simulink model "ACDCMG_sim8"  (R2022a)
settings: Solver=FixedStepAuto  StartTime=0.0  StopTime=0.5  FixedStep=Ts  MaxStep=1e-2  RelTol=1e-3
InitFcn:
  | Set_parameters_R2018
values from neighbouring files (symbols this model uses):
  D_invs = 0.05    [Set_parameters_R2018.m]
  dis11 = 3    [Set_parameters_R2018.m]
  dis12 = 3    [Set_parameters_R2018.m]
  dis2 = 0.2    [Set_parameters_R2018.m]
  dis3 = 0.15    [Set_parameters_R2018.m]
  dis4 = 0.2    [Set_parameters_R2018.m]
  dis5 = 0.25    [Set_parameters_R2018.m]
  dis6 = 0.1    [Set_parameters_R2018.m]
  Fnom = 60    [Set_parameters_R2018.m]
  H_invs = 6    [Set_parameters_R2018.m]
  max_min = 1    [Set_parameters_R2018.m]
  P_Load_3 = S_Load_3* PF_Load_3    (= 7650)    [Set_parameters_R2018.m]
  P_nom_inv = 3e3    (= 3000)    [Set_parameters_R2018.m]
  Pnom_T1 = 1.5e6    (= 1500000)    [Set_parameters_R2018.m]
  Pnom_T2 = 1.5e6    (= 1500000)    [Set_parameters_R2018.m]
  Pnom_T3 = 4e6    (= 4000000)    [Set_parameters_R2018.m]
  Ql_Load_3 = S_Load_3 * sin(acos(PF_Load_3))    [Set_parameters_R2018.m]
  R_Load_9 = (Vnom_prim * 1.35)^2 / P_Load_9    (= 1084.6153125)    [Set_parameters_R2018.m]
  R_Load_DC = Vnom_DC^2/ P_Load_DC    (= 45)    [Set_parameters_R2018.m]
  Rl = 0.17    [Set_parameters_R2018.m]
  Rls = 0.013    [Set_parameters_R2018.m]
  Ts = Ts_Power    (= 6.94444444444e-06)    [Set_parameters_R2018.m]
  Ts_Control = 6*Ts_Power    (= 4.16666666667e-05)    [Set_parameters_R2018.m]
  Ts_Inv = 0.07    [Set_parameters_R2018.m]
  Ts_Power = 1/(24*Fnom)/100    (= 6.94444444444e-06)    [Set_parameters_R2018.m]
  Ts_PV = 0.05    [Set_parameters_R2018.m]
  V1_LL_T3 = 69e3    (= 69000)    [Set_parameters_R2018.m]
  Vmin_mppt = 100    [Set_parameters_R2018.m]
  Vnom_DC = 300    [Set_parameters_R2018.m]
  Vnom_Diesel = 2.4e3    (= 2400)    [Set_parameters_R2018.m]
  Vnom_prim = 13.8e3    (= 13800)    [Set_parameters_R2018.m]
  Vnom_sec = 220    [Set_parameters_R2018.m]
  Vnom_ter_AC_DC = 150    [Set_parameters_R2018.m]
  Xl = 0.3    [Set_parameters_R2018.m]
  Xls = 0.93e-3    (= 0.00093)    [Set_parameters_R2018.m]
undefined symbols (not defined in the file or in its folder): D1, dEgdT, Delta, DiscIntNeverNeededParam, EgRef, fn, gcbh, Ion, k1, Lithium, Rsh_array5pc, sps_rtmsupport, Tref_K, VnInv, VT_ref
libraries: spsCurrentMeasurementLib x40, spsRMSLib x29, spsSeriesRLCBranchLib x23, spsVoltageMeasurementLib x21, spsMeanLib x14, spsThreePhaseVIMeasurementLib x14, powerlib_extras x13, spsThreePhaseSeriesRLCBranchLib x12, spsPower3phInstantaneousLib x10, spsBreakerLib x8, spsControlledVoltageSourceLib x8, spsPowerLib x8
(part 3 of 12)

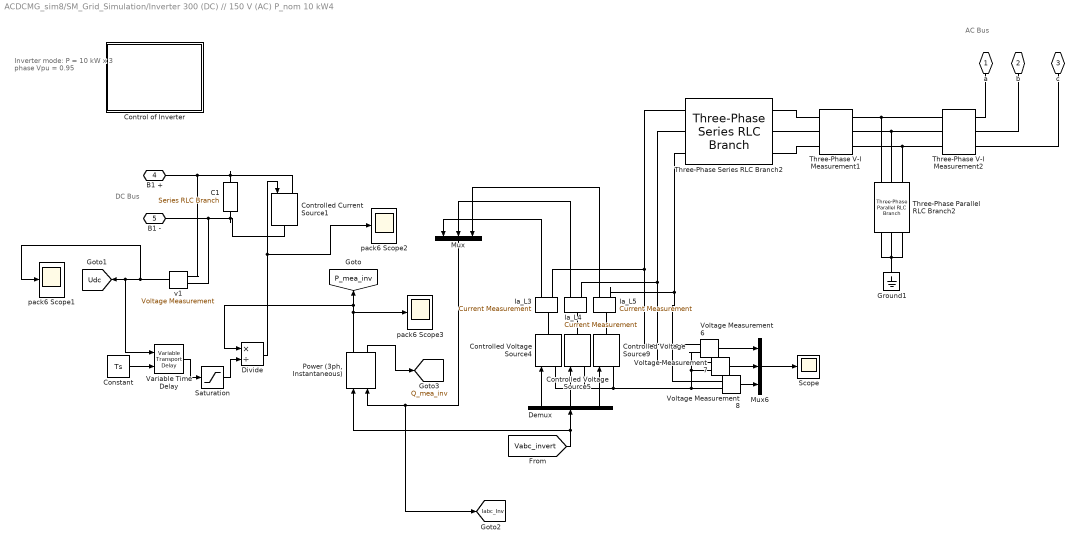
== system ACDCMG_sim8/SM_Grid_Simulation/Inverter 300 (DC) // 150 V (AC) P_nom 10 kW4 ==
  note: DC Bus
  note: AC Bus
  note: Inverter mode:
      |
      | P = 10 kW x 3 phase
      | Vpu = 0.95
  C1 : spsSeriesRLCBranchLib/Series RLC Branch  LConnTagsString=__new0  RConnTagsString=__new0  BranchType=C  Resistance=22.5  Inductance=1e-3  SetiL0=off  InitialCurrent=0  Capacitance=1200e-6  Setx0=on  InitialVoltage=300  Measurements=None
  Constant : Constant  Value=Ts
  Control of Inverter : Subsystem
      mask Display: image('Icons\FPGA.png');
  Controlled Current Source1 : spsControlledCurrentSourceLib/Controlled Current Source  Initialize=on  Source_Type=AC  Amplitude=0  Phase=0  Frequency=0  Measurements=None
  Controlled Voltage Source4 : spsControlledVoltageSourceLib/Controlled Voltage Source  Initialize=off  Source_Type=AC  Amplitude=VnInv*sqrt(2)  Phase=0  Frequency=fn  Measurements=None
  Controlled Voltage Source5 : spsControlledVoltageSourceLib/Controlled Voltage Source  Initialize=off  Source_Type=AC  Amplitude=VnInv*sqrt(2)  Phase=0  Frequency=fn  Measurements=None
  Controlled Voltage Source9 : spsControlledVoltageSourceLib/Controlled Voltage Source  Initialize=off  Source_Type=AC  Amplitude=VnInv*sqrt(2)  Phase=0  Frequency=fn  Measurements=None
  Demux : Demux  Outputs=3
  Divide : Product  Inputs=*/
  Ground1 : spsGroundLib/Ground  LConnTagsString=a
  Ia_L3 : spsCurrentMeasurementLib/Current Measurement  PhasorSimulation=off  OutputType=Complex  PSBequivalent=0
  Ia_L4 : spsCurrentMeasurementLib/Current Measurement  PhasorSimulation=off  OutputType=Complex  PSBequivalent=0
  Ia_L5 : spsCurrentMeasurementLib/Current Measurement  PhasorSimulation=off  OutputType=Complex  PSBequivalent=0
  Mux : Mux  Inputs=3
  Mux6 : Mux  Inputs=3
  "Power (3ph, Instantaneous)" : spsPower3phInstantaneousLib/Power (3ph, Instantaneous)
  Saturation : Saturate  UpperLimit=inf  LowerLimit=0.01
  Scope : Scope
  Three-Phase Parallel RLC Branch2 : spsThreePhaseParallelRLCBranchLib/Three-Phase Parallel RLC Branch  LConnTagsString=A|B|C  RConnTagsString=A|B|C  BranchType=C  Resistance=1  Inductance=1e-3  Capacitance=2.65e-6  Measurements=None
      settings: SourceProductBaseCode=PS
  Three-Phase Series RLC Branch2 : spsThreePhaseSeriesRLCBranchLib/Three-Phase Series RLC Branch  LConnTagsString=A|B|C  RConnTagsString=A|B|C  BranchType=RL  Resistance=0.02  Inductance=1e-2  Capacitance=15.5e-5  Measurements=None
  Three-Phase V-I Measurement1 : spsThreePhaseVIMeasurementLib/Three-Phase V-I Measurement  VoltageMeasurement=phase-to-ground  SetLabelV=on  LabelV=u  Vpu=off  VpuLL=off  CurrentMeasurement=yes  SetLabelI=on  LabelI=i  Ipu=off  Pbase=100e6  Vbase=500e3  OutputType=Complex  PhasorSimulation=off  PSBequivalent=0
  Three-Phase V-I Measurement2 : spsThreePhaseVIMeasurementLib/Three-Phase V-I Measurement  VoltageMeasurement=phase-to-ground  SetLabelV=on  LabelV=Vabc3  Vpu=off  VpuLL=off  CurrentMeasurement=yes  SetLabelI=on  LabelI=Iabc3  Ipu=off  Pbase=100e6  Vbase=500e3  OutputType=Complex  PhasorSimulation=off  PSBequivalent=0
  Variable Time Delay : VariableTransportDelay  MaximumDelay=2*Ts  InitialOutput=Ts
  Voltage Measurement6 : spsVoltageMeasurementLib/Voltage Measurement  PhasorSimulation=off  OutputType=Complex  PSBequivalent=0
  Voltage Measurement7 : spsVoltageMeasurementLib/Voltage Measurement  PhasorSimulation=off  OutputType=Complex  PSBequivalent=0
  Voltage Measurement8 : spsVoltageMeasurementLib/Voltage Measurement  PhasorSimulation=off  OutputType=Complex  PSBequivalent=0
  pack6 Scope1 : Scope
  pack6 Scope2 : Scope
  pack6 Scope3 : Scope
  v1 : spsVoltageMeasurementLib/Voltage Measurement  PhasorSimulation=off  OutputType=Complex  PSBequivalent=0
  "a " : PMIOPort  Tag=PMCPort  Side=Left
  b : PMIOPort  Tag=PMCPort  Port=2  Side=Left
  c : PMIOPort  Tag=PMCPort  Port=3  Side=Left
  B1 + : PMIOPort  Port=4  Side=Right
  B1 - : PMIOPort  Port=5  Side=Right
  tag scope: Iabc_Inv=global, P_mea_inv=global, Q_mea_inv=global, Udc=global
  wires:
  Voltage Measurement8/1 -> Mux6/3
  Mux6/1 -> Scope/1
  Voltage Measurement7/1 -> Mux6/2
  Voltage Measurement6/1 -> Mux6/1
  Demux/3 -> Controlled Voltage Source9/1
  Demux/2 -> Controlled Voltage Source5/1
  Demux/1 -> Controlled Voltage Source4/1
  Ia_L3/1 -> Mux/1
  Ia_L4/1 -> Mux/2
  Ia_L5/1 -> Mux/3
  Mux/1 -> [Iabc_Inv], "Power (3ph, Instantaneous)"/2
  "Power (3ph, Instantaneous)"/1 -> Divide/1, [P_mea_inv], pack6 Scope3/1
  Divide/1 -> pack6 Scope2/1, Controlled Current Source1/1
  [Vabc_invert] -> Demux/1, "Power (3ph, Instantaneous)"/1
  Constant/1 -> Variable Time Delay/2
  v1/1 -> pack6 Scope1/1, Variable Time Delay/1, [Udc]
  Variable Time Delay/1 -> Saturation/1
  Saturation/1 -> Divide/2
  "Power (3ph, Instantaneous)"/2 -> [Q_mea_inv]
  connections:
  Three-Phase V-I Measurement1/RConn1 -- Three-Phase V-I Measurement2/LConn1 -- Three-Phase Parallel RLC Branch2/LConn1
  Three-Phase Parallel RLC Branch2/LConn2 -- Three-Phase V-I Measurement2/LConn2 -- Three-Phase V-I Measurement1/RConn2
  Three-Phase V-I Measurement1/RConn3 -- Three-Phase V-I Measurement2/LConn3 -- Three-Phase Parallel RLC Branch2/LConn3
  Ground1/LConn1 -- Three-Phase Parallel RLC Branch2/RConn3 -- Three-Phase Parallel RLC Branch2/RConn1 -- Three-Phase Parallel RLC Branch2/RConn2
  Ia_L3/RConn1 -- Voltage Measurement6/LConn1 -- Three-Phase Series RLC Branch2/LConn1
  C1/LConn1 -- B1 +/RConn1 -- v1/LConn1 -- Controlled Current Source1/LConn1
  C1/RConn1 -- B1 -/RConn1 -- v1/LConn2 -- Controlled Current Source1/RConn1
  Three-Phase V-I Measurement1/LConn1 -- Three-Phase Series RLC Branch2/RConn1
  Three-Phase V-I Measurement1/LConn2 -- Three-Phase Series RLC Branch2/RConn2
  Three-Phase V-I Measurement1/LConn3 -- Three-Phase Series RLC Branch2/RConn3
  Three-Phase V-I Measurement2/RConn1 -- "a "/RConn1
  Three-Phase V-I Measurement2/RConn2 -- b/RConn1
  Three-Phase V-I Measurement2/RConn3 -- c/RConn1
  Controlled Voltage Source4/LConn1 -- Controlled Voltage Source5/LConn1 -- Controlled Voltage Source9/LConn1 -- Voltage Measurement6/LConn2 -- Voltage Measurement7/LConn2 -- Voltage Measurement8/LConn2
  Ia_L5/RConn1 -- Three-Phase Series RLC Branch2/LConn3 -- Voltage Measurement8/LConn1
  Three-Phase Series RLC Branch2/LConn2 -- Ia_L4/RConn1 -- Voltage Measurement7/LConn1
  Ia_L3/LConn1 -- Controlled Voltage Source4/RConn1
  Ia_L4/LConn1 -- Controlled Voltage Source5/RConn1
  Ia_L5/LConn1 -- Controlled Voltage Source9/RConn1

== system ACDCMG_sim8/SM_Grid_Simulation/Main Grid 69 kV Inf ==
  note: Thevenin equivalent
  69kV 10000 MVA 1 : spsThreePhaseSeriesRLCBranchLib/Three-Phase Series RLC Branch  LConnTagsString=A|B|C  RConnTagsString=A|B|C  BranchType=RL  Resistance=69e3^2/10000e6/10  Inductance=69e3^2/10000e6/(2*pi*60)  Capacitance=1.0  Measurements=None
  Ground1 : spsGroundLib/Ground  LConnTagsString=a
  Programmable Voltage Source1 : spsThreePhaseProgrammableVoltageSourceLib/Three-Phase Programmable Voltage Source  PositiveSequence="[69e3 0  60]"  VariationEntity=None  VariationType=Table of time-amplitude pairs  VariationTypeAlt=Step  VariationStep=-0.3  VariationRate=0.5  VariationMagnitude=0.4  VariationFrequency=2  VariationTiming=[0.1 1.2]  VariationPhaseA=off  Amplitudes=[1]  TimeValues=[0]  HarmonicGeneration=off  HarmonicA=[3 0.2 -25 0]  HarmonicB="[2 0.15  35 2]"  Timing="[0.1  0.6]"  BusType=swing  Pref=500  Qref=0  Qmin=-inf  Qmax=inf
  C : PMIOPort  Side=Right
  B : PMIOPort  Port=2  Side=Right
  A : PMIOPort  Port=3  Side=Right
  connections:
  Programmable Voltage Source1/RConn3 -- 69kV 10000 MVA 1/LConn3
  Ground1/LConn1 -- Programmable Voltage Source1/LConn1
  Programmable Voltage Source1/RConn2 -- 69kV 10000 MVA 1/LConn2
  69kV 10000 MVA 1/LConn1 -- Programmable Voltage Source1/RConn1
  69kV 10000 MVA 1/RConn3 -- C/RConn1
  69kV 10000 MVA 1/RConn2 -- B/RConn1
  69kV 10000 MVA 1/RConn1 -- A/RConn1

== system ACDCMG_sim8/SM_Grid_Simulation/Non Linear AC  Load 9 ==
  Display : Display
  Mean : spsMeanLib/Mean  Freq=100  Vinit=0  Ts=0
  No lineal AC Load 320Kw : spsUniversalBridgeLib/Universal Bridge  Arms=3  SnubberResistance=1e5  SnubberCapacitance=inf  Device=Thyristors  Ron=1e-3  Lon=0  ForwardVoltages="[  0  0  ]"  ForwardVoltage=0  GTOparameters=[ 10e-6 , 20e-6 ]  IGBTparameters=[ 1e-6 , 2e-6 ]  Measurements=None  Measurements_2=None  converterType=Rectifier
  PWM Generator (2-Level) : spsPWMGenerator2LevelLib/PWM Generator (2-Level)  ModulatorType=Three-phase bridge (6 pulses)  ModulatorMode=Unsynchronized  Fc=4080  Pc=0  nF=27  MinMax="[ -1  1 ]"  SamplingTechnique=Natural  ModulatingSignals=on  m=0.8  Freq=Fnom  Phase=-30  Ts=0  ShowCarrierOutport=off
  RL : spsSeriesRLCBranchLib/Series RLC Branch  LConnTagsString=__new0  RConnTagsString=__new0  BranchType=R  Resistance=R_Load_9  Inductance=5e-3  SetiL0=off  InitialCurrent=0  Capacitance=1e-6  Setx0=off  InitialVoltage=0  Measurements=None
  RL1 : spsSeriesRLCBranchLib/Series RLC Branch  LConnTagsString=__new0  RConnTagsString=__new0  BranchType=C  Resistance=1  Inductance=5e-3  SetiL0=off  InitialCurrent=0  Capacitance=10e-6  Setx0=off  InitialVoltage=0  Measurements=None
  "Vdc " : spsVoltageMeasurementLib/Voltage Measurement  Tag=PoWeRsYsTeMmEaSuReMeNt  PhasorSimulation=off  OutputType=Magnitude  PSBequivalent=0
  A : PMIOPort  Tag=PMCPort  Side=Left
  B : PMIOPort  Tag=PMCPort  Port=2  Side=Left
  C : PMIOPort  Tag=PMCPort  Port=3  Side=Left
  wires:
  PWM Generator (2-Level)/1 -> No lineal AC Load 320Kw/1
  "Vdc "/1 -> Mean/1
  Mean/1 -> Display/1
  connections:
  No lineal AC Load 320Kw/RConn1 -- "Vdc "/LConn1 -- RL1/LConn1 -- RL/LConn1
  A/RConn1 -- No lineal AC Load 320Kw/LConn1
  C/RConn1 -- No lineal AC Load 320Kw/LConn3
  B/RConn1 -- No lineal AC Load 320Kw/LConn2
  No lineal AC Load 320Kw/RConn2 -- "Vdc "/LConn2 -- RL1/RConn1 -- RL/RConn1
